simulink model "cruise_contol_sim"  (R2020a)
settings: Solver=ode1  StartTime=0.0  StopTime=50  FixedStep=0.1  RelTol=1e-3
values from neighbouring files (symbols this model uses):
  Crr = 0.002    [Cruise_Control_Script.m]
  Kdrag = 0.5 * rho * Cd * area    (= 0.338390450585)    [Cruise_Control_Script.m]
  Ki = 0.0035    [Cruise_Control_Script.m]
  Kp = 0.4    [Cruise_Control_Script.m]
  mass = 82.7    [Cruise_Control_Script.m]
  MotorRPM = [20 40 60 80 100 120 138 160 178 200 218 240 258 280 298 320]    [Cruise_Control_Script.m]
  MotorTorque = [16.1 14.75 13.85 13.15 12.2 11 9.85 8.2 7.75 6.5 6 5.9 4.2 3.95 3.9 2.1]    [Cruise_Control_Script.m]
  wheelRadius = 0.3302    [Cruise_Control_Script.m]
settings Model: Creator=rafae  LastModifiedBy=rafae

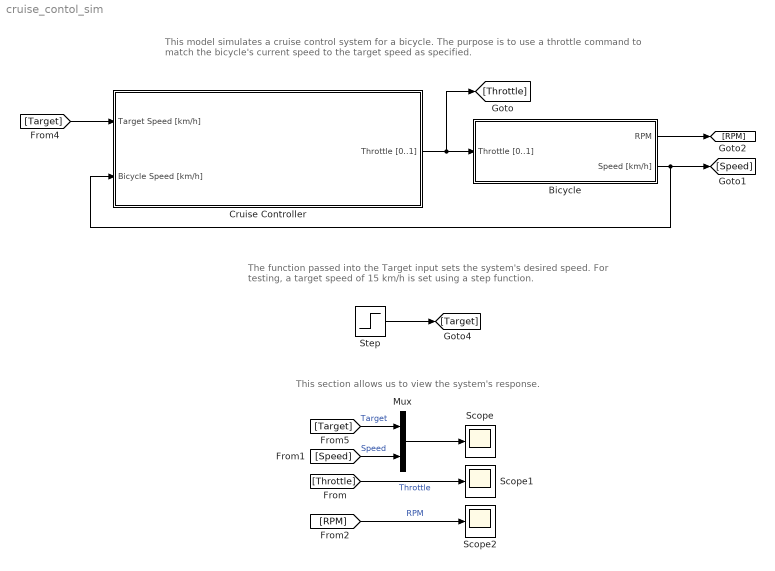
== system cruise_contol_sim ==
  note: The function passed into the Target input sets the system's desired speed.
      | For testing, a target speed of 15 km/h is set using a step function.
  note: This model simulates a cruise control system for a bicycle.
      | The purpose is to use a throttle command to match the bicycle's current speed to the target speed as specified.
  note: This section allows us to view the system's response.
  Bicycle : Subsystem
  Cruise Controller : Subsystem
  Mux : Mux  Inputs=2
  Scope : Scope
  Scope1 : Scope
  Scope2 : Scope
  Step : Step  After=15  SampleTime=0
  wires:
  [Target] -> Cruise Controller/1(Target Speed [km/h])
  Bicycle/2(Speed [km/h]) -> [Speed], Cruise Controller/2(Bicycle Speed [km/h])
  Cruise Controller/1(Throttle [0..1]) -> [Throttle], Bicycle/1(Throttle [0..1])
  Bicycle/1(RPM) -> [RPM]
  [Target] -> Mux/1  "Target"
  [Speed] -> Mux/2  "Speed"
  [Throttle] -> Scope1/1  "Throttle"
  Step/1 -> [Target]
  [RPM] -> Scope2/1  "RPM"
  Mux/1 -> Scope/1

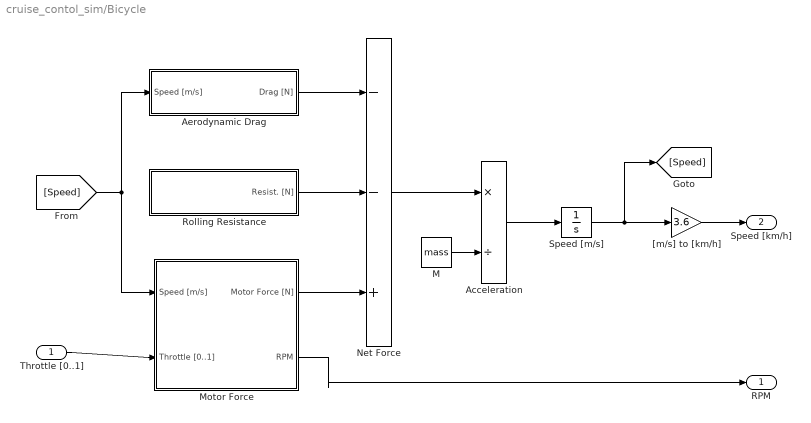
== system cruise_contol_sim/Bicycle ==
  Throttle [0..1] : Inport
  Acceleration : Product  Inputs=*/
  Aerodynamic Drag : Subsystem
  M : Constant  Value=mass
  Motor Force : Subsystem
  Net Force : Sum  Inputs=--+
  Rolling Resistance : Subsystem
  Speed [m/s] : Integrator
  "[m/s] to [km/h]" : Gain  Gain=3.6
  RPM : Outport
  Speed [km/h] : Outport  Port=2
  wires:
  [Speed] -> Aerodynamic Drag/1(Speed [m/s]), Motor Force/1(Speed [m/s])
  Speed [m/s]/1 -> [Speed], "[m/s] to [km/h]"/1
  Motor Force/1(Motor Force [N]) -> Net Force/3
  Net Force/1 -> Acceleration/1
  M/1 -> Acceleration/2
  Aerodynamic Drag/1(Drag [N]) -> Net Force/1
  Throttle [0..1]/1 -> Motor Force/2(Throttle [0..1])
  "[m/s] to [km/h]"/1 -> Speed [km/h]/1
  Acceleration/1 -> Speed [m/s]/1
  Rolling Resistance/1(Resist. [N]) -> Net Force/2
  Motor Force/2(RPM) -> RPM/1

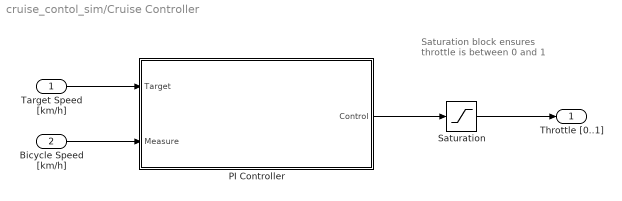
== system cruise_contol_sim/Cruise Controller ==
  note: Saturation block ensures
      | throttle is between 0 and 1
  Target Speed [km/h] : Inport
  Bicycle Speed [km/h] : Inport  Port=2
  PI Controller : Subsystem
  Saturation : Saturate  UpperLimit=1  LowerLimit=0
  Throttle [0..1] : Outport
  wires:
  PI Controller/1(Control) -> Saturation/1
  Target Speed [km/h]/1 -> PI Controller/1(Target)
  Bicycle Speed [km/h]/1 -> PI Controller/2(Measure)
  Saturation/1 -> Throttle [0..1]/1

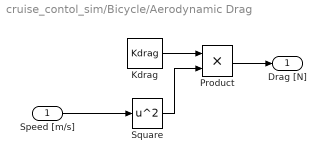
== system cruise_contol_sim/Bicycle/Aerodynamic Drag ==
  Speed [m/s] : Inport
  Kdrag : Constant  Value=Kdrag
  Product : Product
  Square : Math  Operator=square  SaturateOnIntegerOverflow=on
  Drag [N] : Outport
  wires:
  Product/1 -> Drag [N]/1
  Kdrag/1 -> Product/1
  Square/1 -> Product/2
  Speed [m/s]/1 -> Square/1

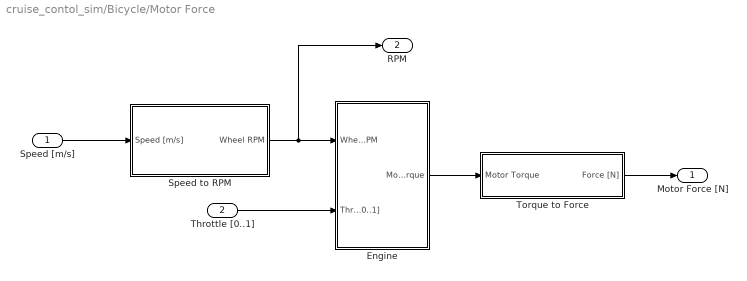
== system cruise_contol_sim/Bicycle/Motor Force ==
  Speed [m/s] : Inport
  Throttle [0..1] : Inport  Port=2
  Engine : Subsystem
  Speed to RPM : Subsystem
  Torque to Force : Subsystem
  Motor Force [N] : Outport
  RPM : Outport  Port=2
  wires:
  Speed to RPM/1(Wheel RPM) -> RPM/1, Engine/1(Wheel RPM)
  Engine/1(Motor Torque) -> Torque to Force/1(Motor Torque)
  Torque to Force/1(Force [N]) -> Motor Force [N]/1
  Throttle [0..1]/1 -> Engine/2(Throttle [0..1])
  Speed [m/s]/1 -> Speed to RPM/1(Speed [m/s])

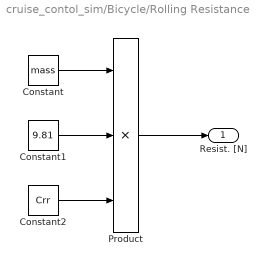
== system cruise_contol_sim/Bicycle/Rolling Resistance ==
  Constant : Constant  Value=mass
  Constant1 : Constant  Value=9.81
  Constant2 : Constant  Value=Crr
  Product : Product  Inputs=3
  Resist. [N] : Outport
  wires:
  Product/1 -> Resist. [N]/1
  Constant1/1 -> Product/2
  Constant/1 -> Product/1
  Constant2/1 -> Product/3

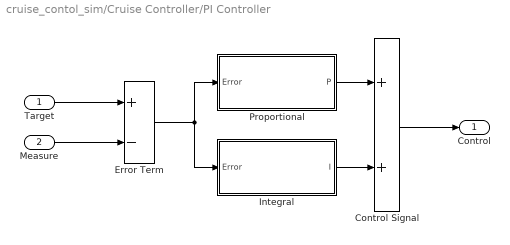
== system cruise_contol_sim/Cruise Controller/PI Controller ==
  Target : Inport
  Measure : Inport  Port=2
  Control Signal : Sum
  Error Term : Sum  Inputs=+-
  Integral : Subsystem
  Proportional : Subsystem
  Control : Outport
  wires:
  Proportional/1(P) -> Control Signal/1
  Control Signal/1 -> Control/1
  Measure/1 -> Error Term/2
  Error Term/1 -> Proportional/1(Error), Integral/1(Error)
  Integral/1(I) -> Control Signal/2
  Target/1 -> Error Term/1

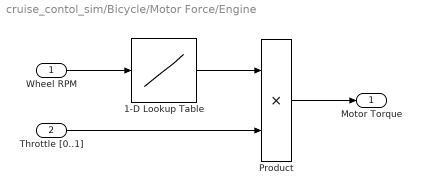
== system cruise_contol_sim/Bicycle/Motor Force/Engine ==
  Wheel RPM : Inport
  Throttle [0..1] : Inport  Port=2
  1-D Lookup Table : Lookup_n-D  NumberOfTableDimensions=1  BreakpointsForDimension1=MotorRPM  Table=MotorTorque  InterpMethod=Cubic spline  InternalRulePriority=Speed  RndMeth=Simplest  InputSameDT=on
  Product : Product
  Motor Torque : Outport
  wires:
  Wheel RPM/1 -> 1-D Lookup Table/1
  Throttle [0..1]/1 -> Product/2
  1-D Lookup Table/1 -> Product/1
  Product/1 -> Motor Torque/1

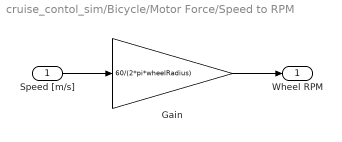
== system cruise_contol_sim/Bicycle/Motor Force/Speed to RPM ==
  Speed [m/s] : Inport
  Gain : Gain  Gain=60/(2*pi*wheelRadius)
  Wheel RPM : Outport
  wires:
  Speed [m/s]/1 -> Gain/1
  Gain/1 -> Wheel RPM/1

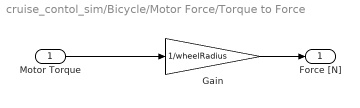
== system cruise_contol_sim/Bicycle/Motor Force/Torque to Force ==
  Motor Torque : Inport
  Gain : Gain  Gain=1/wheelRadius
  Force [N] : Outport
  wires:
  Motor Torque/1 -> Gain/1
  Gain/1 -> Force [N]/1

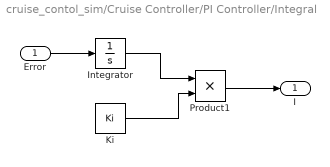
== system cruise_contol_sim/Cruise Controller/PI Controller/Integral ==
  Error : Inport
  Integrator : Integrator
  Ki : Constant  Value=Ki
  Product1 : Product
  I : Outport
  wires:
  Product1/1 -> I/1
  Ki/1 -> Product1/2
  Integrator/1 -> Product1/1
  Error/1 -> Integrator/1

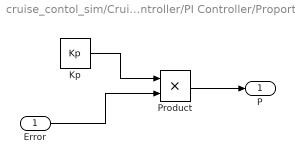
== system cruise_contol_sim/Cruise Controller/PI Controller/Proportional ==
  Error : Inport
  Kp : Constant  Value=Kp
  Product : Product
  P : Outport
  wires:
  Kp/1 -> Product/1
  Error/1 -> Product/2
  Product/1 -> P/1
